simulink model "fxpdemo_sine"  (Simulink 7.6)
settings: Solver=FixedStepDiscrete  SolverMode=SingleTasking  StartTime=0.0  StopTime=inf  FixedStep=.01  MaxStep=0.01  RelTol=1e-3  AbsTol=1e-6
settings Model: MinMaxOverflowLogging=MinMaxAndOverflow  Creator=The MathWorks Inc.  CovMetricSettings=d  ExtModeTrigMode=oneshot  ExtModeArmWhenConnect=off  ExtModeAutoUpdateStatusClock=off
settings DataIOCC: LimitDataPoints=off  SaveOutput=off  SaveTime=off  SignalLoggingName=sigsOut
settings OptimizationCC: InlineParams=on  InlineInvariantSignals=on
settings DebuggingCC: SaveWithParameterizedLinksMsg=none  SignalResolutionControl=TryResolveAllWithWarning  SolverPrmCheckMsg=none  MultiTaskDSMMsg=warning  MultiTaskCondExecSysMsg=none  IntegerOverflowMsg=none  ParameterDowncastMsg=warning  ParameterOverflowMsg=warning  ParameterPrecisionLossMsg=none  StrictBusMsg=None
settings HardwareCC: TargetUnknown=on
settings RTWCC: IncludeERTFirstTime=on

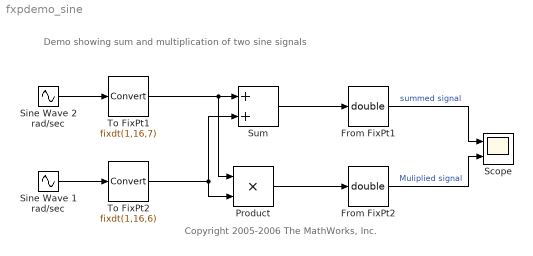
== system fxpdemo_sine ==
  note: Demo showing sum and multiplication of two sine signals
  note: Copyright 2005-2006 The MathWorks, Inc.
  From FixPt1 : DataTypeConversion  OutDataTypeStr=double
  From FixPt2 : DataTypeConversion  OutDataTypeStr=double
  Product : Product  OutDataTypeStr=fixdt(1,16,8)
  Scope : Scope  NumInputPorts=2
      settings: TickLabels=on  TimeRange=10  YMin=-2.5~-1  YMax=2~1
  Sine Wave 1 rad/sec : Sin  SampleTime=0
  Sine Wave 2 rad/sec : Sin  Frequency=2  SampleTime=0
  Sum : Sum  OutDataTypeStr=fixdt(1,16,2)
  To FixPt1 : DataTypeConversion  OutDataTypeStr=fixdt(1,16,7)
  To FixPt2 : DataTypeConversion  OutDataTypeStr=fixdt(1,16,6)
  wires:
  Sine Wave 1 rad/sec/1 -> To FixPt2/1
  Sine Wave 2 rad/sec/1 -> To FixPt1/1
  To FixPt1/1 -> Sum/1, Product/1
  To FixPt2/1 -> Sum/2, Product/2
  From FixPt1/1 -> Scope/1  "summed signal"
  Sum/1 -> From FixPt1/1
  From FixPt2/1 -> Scope/2  "Muliplied signal"
  Product/1 -> From FixPt2/1
